simulink model "simple_active"  (R2022b)
settings: Solver=FixedStepAuto  StartTime=0.0  StopTime=10000  FixedStep=.01  RelTol=1e-3
undefined symbols (not defined in the file): angular, linear
libraries: ros2lib x9
settings Model: Creator=hollis  LastModifiedBy=hollis
settings OptimizationCC: EnhancedBackFolding=on  PassReuseOutputArgsAs=Individual arguments  ZeroExternalMemoryAtStartup=off  ZeroInternalMemoryAtStartup=off  MaxStackSize=64  OptimizeBlockOrder=speed  DifferentSizesBufferReuse=on  OptimizationCustomize=off  EfficientTunableParamExpr=on
settings DebuggingCC: ParameterTunabilityLossMsg=error
settings HardwareCC: ProdBitPerLong=64  ProdLargestAtomicInteger=LongLong  ProdLargestAtomicFloat=Double  ProdLongLongMode=on  ProdHWDeviceType=ARM Compatible->ARM 64-bit (LP64)
settings SFSimCC: MATLABDynamicMemAlloc=off
settings RTWCC: Description=Embedded Coder  SystemTargetFile=ert.tlc  HardwareBoard=Robot Operating System 2 (ROS 2)  TLCOptions="-aInlineSetEventsForThisBaseRateFcn=TLC_FALSE -aSuppressMultiTaskScheduler=TLC_FALSE  -aRateBasedStepFcn=0"  TemplateMakefile=ert_default_tmf  Toolchain=Colcon Tools  BuildConfiguration=Faster Runs  TargetLang=C++
settings CodeAppCC: ForceParamTrailComments=on  IgnoreCustomStorageClasses=off  OperatorAnnotations=on  SimulinkDataObjDesc=on  SFDataObjDesc=on  InsertBlockDesc=on
settings ERTTargetCC: CodeInterfacePackaging=C++ class  SupportVariableSizeSignals=on  RootIOFormat=Structure reference

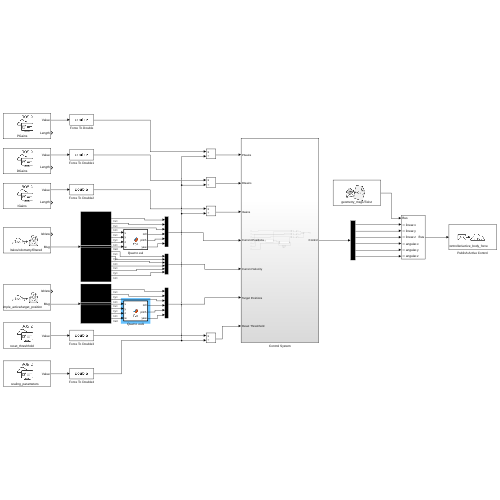
[thumbnail: Simulink's stored preview of the top-level diagram]
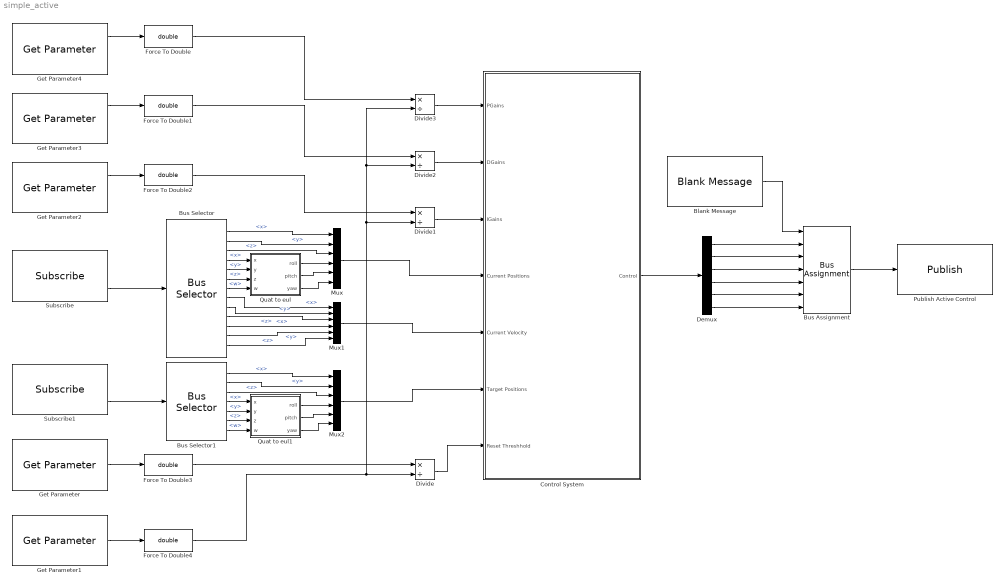
== system simple_active ==
  Blank Message : ros2lib/Blank Message  messageClass=Message  entityType=geometry_msgs/Twist  messageType=geometry_msgs/Twist  SampleTime=inf
      settings: LibrarySourceBlock=roslib/ROS 2/Blank Message
  Bus Assignment : BusAssignment  AssignedSignals=linear.x,linear.y,linear.z,angular.x,angular.y,angular.z
  Bus Selector : BusSelector  OutputSignals=pose.pose.position.x,pose.pose.position.y,pose.pose.position.z,pose.pose.orientation.x,pose.pose.orientation.y,pose.pose.orientation.z,pose.pose.orientation.w,twist.twist.linear.x,twist.twist.linear.y,twist.twist.linear.z,twist.twist.angular.x,twist.twist.angular.y,twist.twist.angular.z
  Bus Selector1 : BusSelector  OutputSignals=position.x,position.y,position.z,orientation.x,orientation.y,orientation.z,orientation.w
  Control System : Subsystem
  Demux : Demux  Outputs=6
  Divide{,1..3} (4 alike) : Product  Inputs=*/
  Force To Double{,1..4} (5 alike) : DataTypeConversion  OutDataTypeStr=double  SaturateOnIntegerOverflow=off  RndMeth=Floor
  Get Parameter : ros2lib/Get Parameter  ParameterName=reset_threshhold  ParameterType=int64  ParameterMaxArrayLength=16  ParameterInitialValue=100000  SampleTime=-1  ModelName=simple_active  BlockId=ParamGet_simple_active_43
      settings: LibrarySourceBlock=roslib/ROS 2/Get Parameter
  Get Parameter1 : ros2lib/Get Parameter  ParameterName=scaling_parameters  ParameterType=int64  ParameterMaxArrayLength=16  ParameterInitialValue=1000000  SampleTime=-1  ModelName=simple_active  BlockId=ParamGet_simple_active_44
      settings: LibrarySourceBlock=roslib/ROS 2/Get Parameter
  Get Parameter2 : ros2lib/Get Parameter  ParameterName=IGains  ParameterType=int64[]  ParameterMaxArrayLength=6  ParameterInitialValue=[0,0,0,0,0,0]  SampleTime=-1  ModelName=simple_active  BlockId=ParamGet_simple_active_46
      settings: LibrarySourceBlock=roslib/ROS 2/Get Parameter
  Get Parameter3 : ros2lib/Get Parameter  ParameterName=DGains  ParameterType=int64[]  ParameterMaxArrayLength=6  ParameterInitialValue=[0,0,0,0,0,0]  SampleTime=-1  ModelName=simple_active  BlockId=ParamGet_simple_active_47
      settings: LibrarySourceBlock=roslib/ROS 2/Get Parameter
  Get Parameter4 : ros2lib/Get Parameter  ParameterName=PGains  ParameterType=int64[]  ParameterMaxArrayLength=6  ParameterInitialValue=[0,0,0,0,0,0]  SampleTime=-1  ModelName=simple_active  BlockId=ParamGet_simple_active_48
      settings: LibrarySourceBlock=roslib/ROS 2/Get Parameter
  Mux : Mux  Inputs=6
  Mux1 : Mux  Inputs=6
  Mux2 : Mux  Inputs=6
  Publish Active Control : ros2lib/Publish  topicSource=Specify your own  topic=/talos/controller/active_body_force  messageType=geometry_msgs/Twist  QOSHistory=Keep last  QOSDepth=1  QOSReliability=Reliable  QOSDurability=Volatile
      settings: LibrarySourceBlock=roslib/ROS 2/Publish
  Quat to eul : MATLAB Function  TreatAsAtomicUnit=on
  Quat to eul1 : MATLAB Function  TreatAsAtomicUnit=on
  Subscribe : ros2lib/Subscribe  topicSource=Specify your own  topic=/talos/odometry/filtered  messageType=nav_msgs/Odometry  sampleTime=-1  QOSHistory=Keep last  QOSDepth=1  QOSReliability=Reliable  QOSDurability=Volatile
      settings: LibrarySourceBlock=roslib/ROS 2/Subscribe
  Subscribe1 : ros2lib/Subscribe  topicSource=Specify your own  topic=/talos/simple_active/target_position  messageType=geometry_msgs/Pose  sampleTime=-1  QOSHistory=Keep last  QOSDepth=1  QOSReliability=Reliable  QOSDurability=Volatile
      settings: LibrarySourceBlock=roslib/ROS 2/Subscribe
  wires:
  Subscribe/2 -> Bus Selector/1
  Bus Selector/4 -> Quat to eul/1(x)  "<x>"
  Bus Selector/5 -> Quat to eul/2(y)  "<y>"
  Bus Selector/6 -> Quat to eul/3(z)  "<z>"
  Bus Selector/7 -> Quat to eul/4(w)  "<w>"
  Quat to eul/3(yaw) -> Mux/6
  Quat to eul/2(pitch) -> Mux/5
  Quat to eul/1(roll) -> Mux/4
  Bus Selector/1 -> Mux/1  "<x>"
  Bus Selector/2 -> Mux/2  "<y>"
  Bus Selector/3 -> Mux/3  "<z>"
  Bus Selector/9 -> Mux1/2  "<y>"
  Bus Selector/8 -> Mux1/1  "<x>"
  Bus Selector/10 -> Mux1/3  "<z>"
  Bus Selector/11 -> Mux1/4  "<x>"
  Bus Selector/12 -> Mux1/5  "<y>"
  Bus Selector/13 -> Mux1/6  "<z>"
  Mux/1 -> Control System/4(Current Positions)
  Mux1/1 -> Control System/5(Current Velocity)
  Subscribe1/2 -> Bus Selector1/1
  Quat to eul1/1(roll) -> Mux2/4
  Quat to eul1/3(yaw) -> Mux2/6
  Quat to eul1/2(pitch) -> Mux2/5
  Get Parameter/1 -> Force To Double3/1
  Get Parameter1/1 -> Force To Double4/1
  Divide/1 -> Control System/7(Reset Threshhold)
  Get Parameter2/1 -> Force To Double2/1
  Get Parameter3/1 -> Force To Double1/1
  Get Parameter4/1 -> Force To Double/1
  Blank Message/1 -> Bus Assignment/1
  Demux/1 -> Bus Assignment/2
  Demux/2 -> Bus Assignment/3
  Demux/3 -> Bus Assignment/4
  Demux/4 -> Bus Assignment/5
  Demux/5 -> Bus Assignment/6
  Demux/6 -> Bus Assignment/7
  Control System/1(Control) -> Demux/1
  Bus Assignment/1 -> Publish Active Control/1
  Force To Double3/1 -> Divide/1
  Force To Double4/1 -> Divide3/2, Divide2/2, Divide1/2, Divide/2
  Mux2/1 -> Control System/6(Target Positions)
  Bus Selector1/1 -> Mux2/1  "<x>"
  Bus Selector1/2 -> Mux2/2  "<y>"
  Bus Selector1/4 -> Quat to eul1/1(x)  "<x>"
  Bus Selector1/5 -> Quat to eul1/2(y)  "<y>"
  Bus Selector1/6 -> Quat to eul1/3(z)  "<z>"
  Bus Selector1/7 -> Quat to eul1/4(w)  "<w>"
  Bus Selector1/3 -> Mux2/3  "<z>"
  Divide3/1 -> Control System/1(PGains)
  Divide2/1 -> Control System/2(DGains)
  Divide1/1 -> Control System/3(IGains)
  Force To Double2/1 -> Divide1/1
  Force To Double1/1 -> Divide2/1
  Force To Double/1 -> Divide3/1

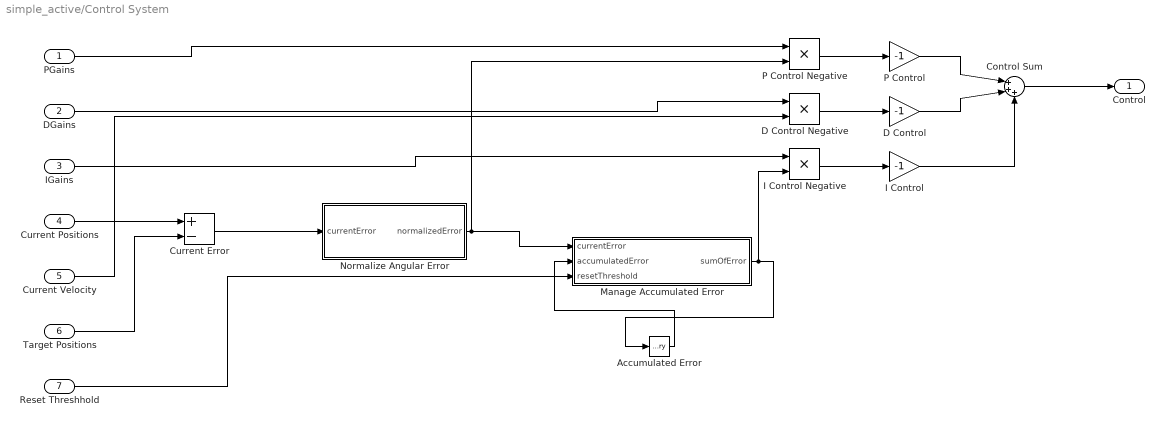
== system simple_active/Control System ==
  PGains : Inport
  DGains : Inport  Port=2
  IGains : Inport  Port=3
  Current Positions : Inport  Port=4
  Current Velocity : Inport  Port=5
  Target Positions : Inport  Port=6
  Reset Threshhold : Inport  Port=7
  Accumulated Error : Memory
  Control Sum : Sum  Inputs=|+++
  Current Error : Sum  Inputs=+-
  D Control : Gain  Gain=-1
  D Control Negative : Product
  I Control : Gain  Gain=-1
  I Control Negative : Product
  Manage Accumulated Error : MATLAB Function  TreatAsAtomicUnit=on
  Normalize Angular Error : MATLAB Function  TreatAsAtomicUnit=on
  P Control : Gain  Gain=-1
  P Control Negative : Product
  Control : Outport
  wires:
  Reset Threshhold/1 -> Manage Accumulated Error/3(resetThreshold)
  Current Positions/1 -> Current Error/1
  DGains/1 -> D Control Negative/1
  I Control/1 -> Control Sum/3
  Current Velocity/1 -> D Control Negative/2
  PGains/1 -> P Control Negative/1
  P Control/1 -> Control Sum/1
  D Control Negative/1 -> D Control/1
  P Control Negative/1 -> P Control/1
  Accumulated Error/1 -> Manage Accumulated Error/2(accumulatedError)
  D Control/1 -> Control Sum/2
  Manage Accumulated Error/1(sumOfError) -> Accumulated Error/1, I Control Negative/2
  I Control Negative/1 -> I Control/1
  Control Sum/1 -> Control/1
  Target Positions/1 -> Current Error/2
  IGains/1 -> I Control Negative/1
  Current Error/1 -> Normalize Angular Error/1(currentError)
  Normalize Angular Error/1(normalizedError) -> P Control Negative/2, Manage Accumulated Error/1(currentError)

== matlab function simple_active/Quat to eul ==
  data: x input; roll output; y input; z input; w input; pitch output; yaw output
function [roll, pitch, yaw] = fcn(x,y,z,w)

%convert the quaternion to euler
euler = quat2eul([w,x,y,z]);

roll = euler(3);
pitch = euler(2);
yaw = euler(1);

== matlab function simple_active/Control System/Manage Accumulated Error ==
  data: currentError input; sumOfError output; accumulatedError input; resetThreshold input
function sumOfError = fcn(currentError, accumulatedError, resetThreshold)

sum = zeros(1,6);

%check each degree of freedom
for i = 1:6
    sum(i) = accumulatedError(i) + currentError(i);

    if(currentError(i) > resetThreshold)
        sum(i) = 0;
    end

    %reset if nan
    if(isnan(currentError(i)))
        sum(i) = 0;
    end

end

sumOfError = sum;

== matlab function simple_active/Control System/Normalize Angular Error ==
  data: currentError input; normalizedError output
function normalizedError = fcn(currentError)

normalized = zeros(1,6);

normalized(1) = currentError(1);
normalized(2) = currentError(2);
normalized(3) = currentError(3);

%each angular degree of freedom
for i=4:6
    %normalize all error to between postive and negative 180
    normalized(i) = mod(currentError(i) + pi, 2 * pi) - pi;
end

normalizedError = normalized;

== matlab function simple_active/Quat to eul1 ==
  data: x input; roll output; y input; z input; w input; pitch output; yaw output
function [roll, pitch, yaw] = fcn(x,y,z,w)

%convert the quaternion to euler
euler = quat2eul([w,x,y,z]);

roll = euler(3);
pitch = euler(2);
yaw = euler(1);

if(isnan(roll))
   roll = 0;
   pitch = 0;
   yaw = 0;
end
